simulink model "harmonic_analysis"  (R2016a)
settings: Solver=VariableStepAuto  StartTime=0.0  StopTime=Tfinal  RelTol=1e-3
values from neighbouring files (symbols this model uses):
  Ts = 100e-9    (= 1e-07)    [for_plots.m]
libraries: powerlib x1
settings Model: Creator=mesutto  LastModifiedBy=mesutto

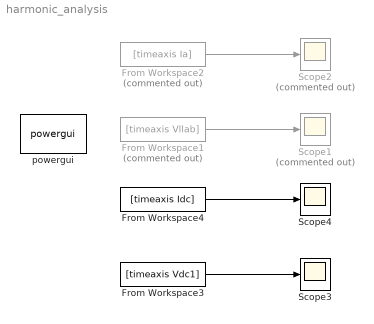
== system harmonic_analysis ==
  From Workspace1 : FromWorkspace  Commented=on  VariableName=[timeaxis Vllab]  OutDataTypeStr=double  SampleTime=Ts
  From Workspace2 : FromWorkspace  Commented=on  VariableName=[timeaxis Ia]  OutDataTypeStr=double  SampleTime=Ts
  From Workspace3 : FromWorkspace  VariableName=[timeaxis Vdc1]  OutDataTypeStr=double  SampleTime=Ts
  From Workspace4 : FromWorkspace  VariableName=[timeaxis Idc]  OutDataTypeStr=double  SampleTime=Ts
  Scope1 : Scope  Commented=on
  Scope2 : Scope  Commented=on
  Scope3 : Scope
  Scope4 : Scope
  powergui : powerlib/powergui  Priority=1  SimulationMode=Discrete  SolverType=Tustin/Backward Euler (TBE)  SampleTime=Ts  frequency=60  SPID=off  DisableSnubberDevices=off  DisableRonSwitches=off  DisableVfSwitches=off  SwTol=0  DisplayEquations=off  Interpol=off  ExternalGateDelay=off  methode=off  Ts=10  FunctionMessages=off  echomessages=off  HookPort=off  EnableUseOfTLC=off  x0status=blocks  frequencyindice=60  Pbase=100e6  ErrMax=1e-4  Iterations=50  UnitsV=kV  UnitsW=MW  buscounter=0  RestoreLinks=warning  ResistiveCurrentMeasurement=off  Frange=[0:2:500]  Ylog=off  Xlog=on  ShowGrid=off  save=off  variable=ZData  structure=Vdc1  ZoomFFT=off  StartTime=0  cycles=2  DisplayStyle=5  fundamental=50  FreqAxis=off  MaxFrequency=200000  frequencyindicesteady=1  RmsSteady=1  display=off
  wires:
  From Workspace2/1 -> Scope2/1
  From Workspace1/1 -> Scope1/1
  From Workspace4/1 -> Scope4/1
  From Workspace3/1 -> Scope3/1
